simulink model "Model"  (R2021a)
settings: Solver=VariableStepAuto  StartTime=0.0  StopTime=10.0  RelTol=1e-3
undefined symbols (not defined in the file or in its folder): g0, M
libraries: shared6dof x1
settings Model: Creator=Adam  LastModifiedBy=Adam

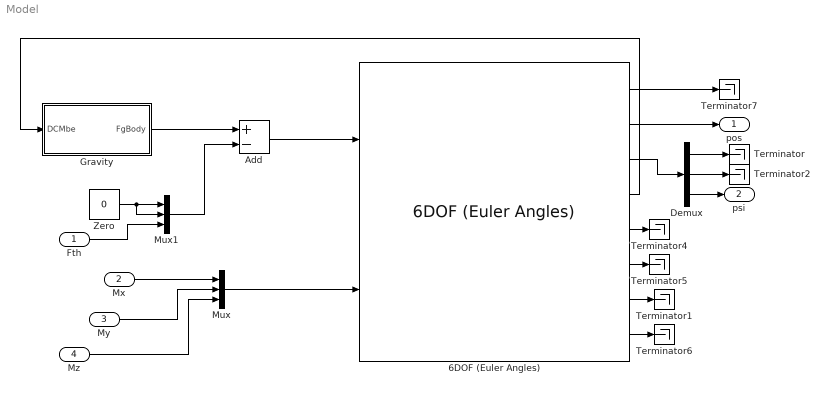
== system Model ==
  Fth : Inport
  Mx : Inport  Port=2
  My : Inport  Port=3
  Mz : Inport  Port=4
  6DOF (Euler Angles) : shared6dof/6DOF (Euler Angles)  units=Metric (MKS)  mtype=Fixed  rep=Euler Angles  xme_0=x0  Vm_0=[0 0 0]  eul_0=[0 0 0]  pm_0=[0 0 0]  mass_0=M  mass_e=0.5  mass_f=2.0  inertia=Ib  inertia_e=eye(3)  inertia_f=2*eye(3)  k_quat=1.0  vre_flag=on  abi_flag=off  aMode=0  xme_statename='Xe'  Vm_statename='Ve'  eul_statename='Euler'  quat_statename=''  pm_statename='Omega'  mass_statename=''
      settings: SourceProductBaseCode=AE,PW,DR,MT,UV,VE
  Add : Sum  Inputs=+-
  Demux : Demux  Outputs=3
  "Gravity " : Subsystem
  Mux : Mux  Inputs=3
  Mux1 : Mux  Inputs=3
  Terminator{,1..2,4..7} (7 alike) : Terminator
  Zero : Constant  Value=0  OutDataTypeStr=Inherit: Inherit via back propagation
  pos : Outport
  psi : Outport  Port=2
  wires:
  6DOF (Euler Angles)/7 -> Terminator1/1
  Zero/1 -> Mux1/2, Mux1/1
  "Gravity "/1(FgBody) -> Add/1
  6DOF (Euler Angles)/4 -> "Gravity "/1(DCMbe)
  Mux1/1 -> Add/2
  Add/1 -> 6DOF (Euler Angles)/1
  6DOF (Euler Angles)/2 -> pos/1
  6DOF (Euler Angles)/3 -> Demux/1
  Demux/1 -> Terminator/1
  Demux/2 -> Terminator2/1
  Demux/3 -> psi/1
  6DOF (Euler Angles)/5 -> Terminator4/1
  6DOF (Euler Angles)/6 -> Terminator5/1
  6DOF (Euler Angles)/1 -> Terminator7/1
  6DOF (Euler Angles)/8 -> Terminator6/1
  Fth/1 -> Mux1/3
  Mux/1 -> 6DOF (Euler Angles)/2
  Mx/1 -> Mux/1
  My/1 -> Mux/2
  Mz/1 -> Mux/3

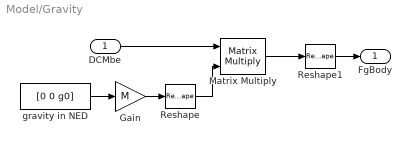
== system Model/Gravity  ==
  DCMbe : Inport
  Gain : Gain  Gain=M
  Matrix Multiply : Product  Multiplication=Matrix(*)
  Reshape : Reshape  OutputDimensionality=Column vector (2-D)
  Reshape1 : Reshape
  gravity in NED : Constant  Value=[0 0 g0]
  FgBody : Outport
  wires:
  gravity in NED/1 -> Gain/1
  Reshape/1 -> Matrix Multiply/2
  Matrix Multiply/1 -> Reshape1/1
  DCMbe/1 -> Matrix Multiply/1
  Gain/1 -> Reshape/1
  Reshape1/1 -> FgBody/1
